simulink model "ISTrain2024"  (R2025a)
settings: Solver=ode4  StartTime=0.0  StopTime=StopTime  FixedStep=StepSize  RelTol=1e-3
undefined symbols (not defined in the file or in its folder): Crr, G, g, LM, LR, m_loco, maxID, maxIQ, maxTorque, mech_eff, Pp, Rr, rw
libraries: slpidlib x3
settings Model: Creator=rafae  LastModifiedBy=mmeni

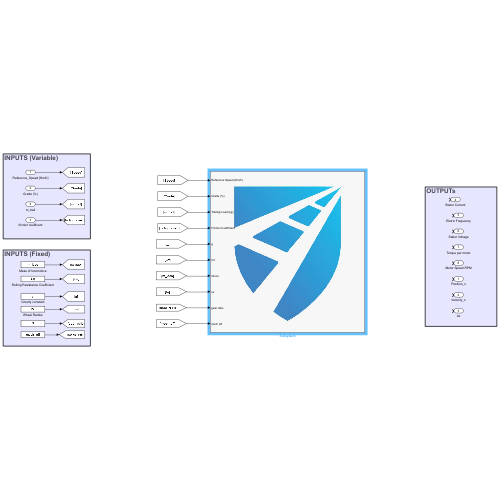
[thumbnail: Simulink's stored preview of the top-level diagram]
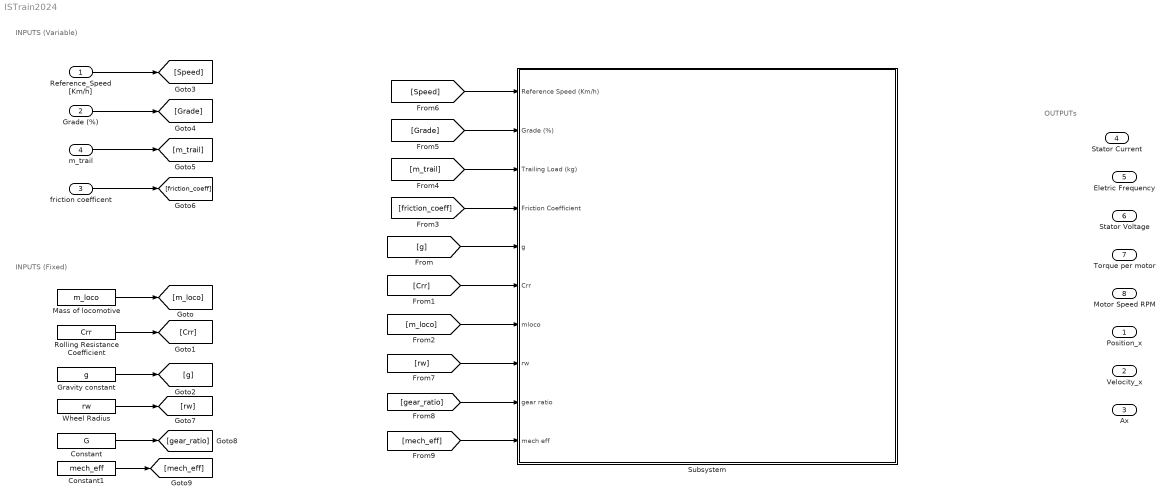
== system ISTrain2024 ==
  note: OUTPUTs
  note: INPUTS (Variable)
  note: INPUTS (Fixed)
  Reference_Speed [Km/h] : Inport
  Grade (%) : Inport  Port=2
  friction coefficent : Inport  Port=3
  m_trail : Inport  Port=4
  Constant : Constant  Value=G
  Constant1 : Constant  Value=mech_eff
  Gravity constant : Constant  Value=g
  Mass of locomotive : Constant  Value=m_loco
  Rolling Resistance Coefficient : Constant  Value=Crr
  Subsystem : Subsystem
      mask Display: image('ist_train_logo.jpg');
  Wheel Radius : Constant  Value=rw
  Position_x : Outport
  Velocity_x : Outport  Port=2
  Ax : Outport  Port=3
  Stator Current : Outport  Port=4
  Eletric Frequency : Outport  Port=5
  Stator Voltage : Outport  Port=6
  Torque per motor : Outport  Port=7
  Motor Speed RPM : Outport  Port=8
  wires:
  Reference_Speed [Km/h]/1 -> [Speed]
  Grade (%)/1 -> [Grade]
  m_trail/1 -> [m_trail]
  friction coefficent/1 -> [friction_coeff]
  Mass of locomotive/1 -> [m_loco]
  Rolling Resistance Coefficient/1 -> [Crr]
  Gravity constant/1 -> [g]
  [g] -> Subsystem/5(g)
  [Crr] -> Subsystem/6(Crr)
  [m_loco] -> Subsystem/7(mloco)
  [friction_coeff] -> Subsystem/4(Friction Coefficient)
  [m_trail] -> Subsystem/3(Trailing Load (kg))
  [Grade] -> Subsystem/2(Grade (%))
  [Speed] -> Subsystem/1(Reference Speed (Km/h))
  Wheel Radius/1 -> [rw]
  [rw] -> Subsystem/8(rw)
  Constant/1 -> [gear_ratio]
  [gear_ratio] -> Subsystem/9(gear ratio)
  Constant1/1 -> [mech_eff]
  [mech_eff] -> Subsystem/10(mech eff)

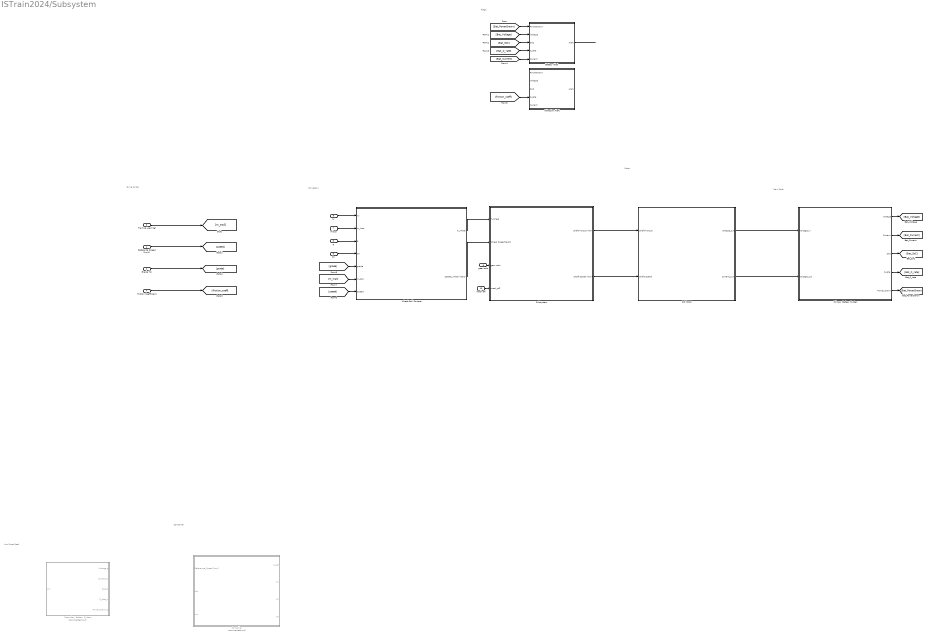
== system ISTrain2024/Subsystem ==
  note: Auxilioar Pack
  note: Drive Cycle
  note: Drivetrain
  note: Motor
  note: Flags
  note: Controller
  note: Main Pack
  Reference Speed (Km/h) : Inport
  Grade (%) : Inport  Port=2
  Trailing Load (kg) : Inport  Port=3
  Friction Coefficient : Inport  Port=4
  g : Inport  Port=5
  Crr : Inport  Port=6
  mloco : Inport  Port=7
  rw : Inport  Port=8
  gear ratio : Inport  Port=9
  mech eff : Inport  Port=10
  Adhesion Alert : Subsystem
      mask Display: image('hazard.jpg');
  Battery Alert : Subsystem
      mask Display: image('hazard.jpg');
  Controller : Subsystem  Commented=on
      mask Display: image('motor controller.jpeg');
  DC Motot : Subsystem
      mask Display: image('motor.jpg');
  Primary Battery Systen : Subsystem
      mask Display: image('battery system.png');
  Secondary Battery System : Subsystem  Commented=on
      mask Display: image('battery system.png');
  Subsystem : Subsystem
      mask Display: image('gear_system.png');
  Wheel-Rail Contact : Subsystem
      mask Display: image('wheel_train.jpg');
  wires:
  Primary Battery Systen/1(Voltage) -> [Bat_Voltage]
  Primary Battery Systen/2(Current) -> [Bat_Current]
  Primary Battery Systen/3(SoC) -> [Bat_SoC]
  Primary Battery Systen/5(Power_drawn) -> [Bat_PowerDrawn]
  Primary Battery Systen/4(C_rate) -> [Bat_C_rate]
  [Bat_Current] -> Battery Alert/5(Current)
  [Bat_C_rate] -> Battery Alert/4(C_rate)
  [Bat_SoC] -> Battery Alert/3(SoC)
  [Bat_Voltage] -> Battery Alert/2(Voltage)
  [Bat_PowerDrawn] -> Battery Alert/1(PowerDrawn)
  Battery Alert/1(Alert) -> ?
  Grade (%)/1 -> [grade]
  Trailing Load (kg)/1 -> [m_trail]
  Friction Coefficient/1 -> [friction_coeff]
  Reference Speed (Km/h)/1 -> [speed]
  g/1 -> Wheel-Rail Contact/3(g)
  Crr/1 -> Wheel-Rail Contact/4(Crr)
  mloco/1 -> Wheel-Rail Contact/2(m_loco)
  [friction_coeff] -> Adhesion Alert/4(C_rate)
  [grade] -> Wheel-Rail Contact/5(grade)
  [m_trail] -> Wheel-Rail Contact/6(m_trail)
  [speed] -> Wheel-Rail Contact/7(Speed)
  rw/1 -> Wheel-Rail Contact/1(rw)
  Wheel-Rail Contact/1(T_wheel) -> Subsystem/1(T_wheel)
  Wheel-Rail Contact/2(Speed_wheel (rad/s)) -> Subsystem/2(Wheel Speed(rad/s))
  gear ratio/1 -> Subsystem/3(gear ratio)
  mech eff/1 -> Subsystem/4(mech_eff)
  Subsystem/1(Shaft Torque (Nm)) -> DC Motot/1(Shaft Torque)
  Subsystem/2(Shaft Speed (rpm)) -> DC Motot/2(Shaft Speed)
  DC Motot/1(Voltage_out) -> Primary Battery Systen/1(Voltage_in)
  DC Motot/2(Current_out) -> Primary Battery Systen/2(Voltage_out)

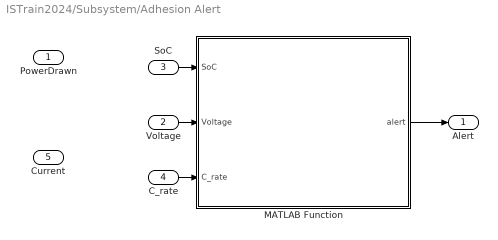
== system ISTrain2024/Subsystem/Adhesion Alert ==
  PowerDrawn : Inport
  Voltage : Inport  Port=2
  SoC : Inport  Port=3
  C_rate : Inport  Port=4
  Current : Inport  Port=5
  MATLAB Function : MATLAB Function  TreatAsAtomicUnit=on
  Alert : Outport
  wires:
  Voltage/1 -> MATLAB Function/2(Voltage)
  SoC/1 -> MATLAB Function/1(SoC)
  MATLAB Function/1(alert) -> Alert/1
  C_rate/1 -> MATLAB Function/3(C_rate)

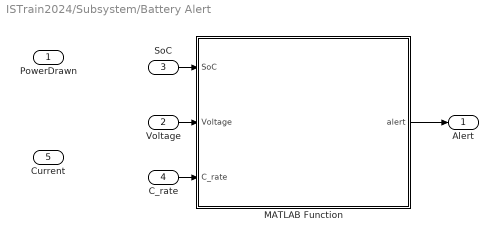
== system ISTrain2024/Subsystem/Battery Alert ==
  PowerDrawn : Inport
  Voltage : Inport  Port=2
  SoC : Inport  Port=3
  C_rate : Inport  Port=4
  Current : Inport  Port=5
  MATLAB Function : MATLAB Function  TreatAsAtomicUnit=on
  Alert : Outport
  wires:
  Voltage/1 -> MATLAB Function/2(Voltage)
  SoC/1 -> MATLAB Function/1(SoC)
  MATLAB Function/1(alert) -> Alert/1
  C_rate/1 -> MATLAB Function/3(C_rate)

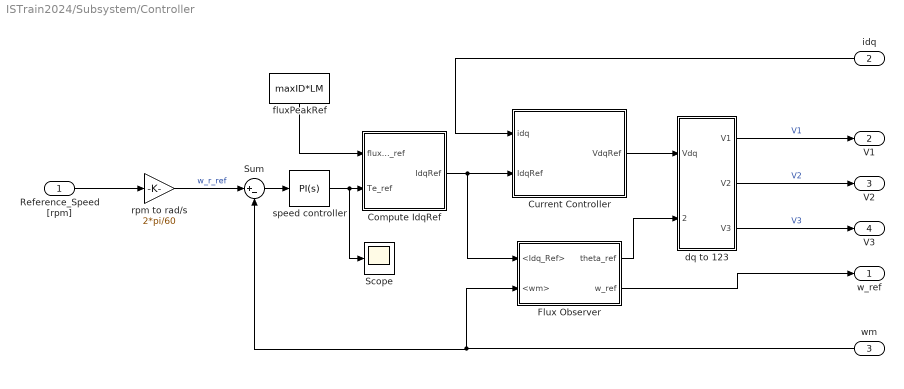
== system ISTrain2024/Subsystem/Controller ==
  Reference_Speed [rpm] : Inport
  idq : Inport  Port=2
  wm : Inport  Port=3
  Compute IdqRef : Subsystem
  Current Controller : Subsystem
  Flux Observer : Subsystem
  Scope : Scope
      settings: ActiveDisplayYMinimum=-8.125  ActiveDisplayYMaximum=73.125
  Sum : Sum  Inputs=|+-
  dq to 123 : Subsystem
  fluxPeakRef : Constant  Value=maxID*LM
  rpm to rad/s : Gain  Gain=2*pi/60
  speed controller : slpidlib/PID Controller  Controller=PI  Form=Parallel  TimeDomain=Continuous-time  UseExternalTs=off  SampleTime=-1  IntegratorMethod=Forward Euler  FilterMethod=Forward Euler  ControllerParametersSource=internal  P=50  I=100  UseKiTs=off  D=0  UseExternalDerivativeSource=off  N=100  UseFilter=on  TunerSelectOption=Transfer Function Based (PID Tuner App)  InitialConditionSource=internal  InitialConditionForIntegrator=0  InitialConditionForFilter=0  DifferentiatorICPrevScaledInput=0  ExternalReset=none  TrackingMode=off  Kt=1  LimitOutput=on  SatLimitsSource=internal  UpperSaturationLimit=maxTorque  LowerSaturationLimit=-maxTorque  LinearizeAsGain=on  AntiWindupMode=back-calculation  Kb=500  LimitIntegrator=off  UpperIntegratorSaturationLimit=inf  LowerIntegratorSaturationLimit=-inf  POutMin=[]  POutMax=[]  IOutMin=[]  IOutMax=[]  DOutMin=[]  DOutMax=[]  NOutMin=[]  NOutMax=[]  SumOutMin=[]  SumOutMax=[]  SaturationOutMin=[]  SaturationOutMax=[]  PParamMin=[]  PParamMax=[]  IParamMin=[]  IParamMax=[]  DParamMin=[]  DParamMax=[]  NParamMin=[]  NParamMax=[]  KbParamMin=[]  KbParamMax=[]  KtParamMin=[]  KtParamMax=[]  KbOutMin=[]  KbOutMax=[]  KtOutMin=[]  KtOutMax=[]  IntegratorOutMin=[]  IntegratorOutMax=[]  FilterOutMin=[]  FilterOutMax=[]  SumI1OutMin=[]  SumI1OutMax=[]  SumI2OutMin=[]  SumI2OutMax=[]  SumI3OutMin=[]  SumI3OutMax=[]  SumI4OutMin=[]  SumI4OutMax=[]  SumDOutMin=[]  SumDOutMax=[]  DifferentiatorOutMin=[]  DifferentiatorOutMax=[]  FilterDiffOutCoefMin=[]  FilterDiffOutCoefMax=[]  ReciprocalOutMin=[]  ReciprocalOutMax=[]  SumDenOutMin=[]  SumDenOutMax=[]  SumNumOutMin=[]  SumNumOutMax=[]  DivideOutMin=[]  DivideOutMax=[]  UdiffTsProdOutMin=[]  UdiffTsProdOutMax=[]  NTsProdOutMin=[]  NTsProdOutMax=[]  UintegralTsProdOutMin=[]  UintegralTsProdOutMax=[]  UngainTsProdOutMin=[]  UngainTsProdOutMax=[]  ClampingZeroOutDataTypeStr=Inherit: Inherit via back propagation  ClampingZeroOutMin=[]  ClampingZeroOutMax=[]  FilterDenConstantOutDataTypeStr=Inherit: Inherit via back propagation  FilterDenConstantOutMin=[]  FilterDenConstantOutMax=[]  PCopyOutDataTypeStr=Inherit: Inherit via back propagation  PCopyOutMin=[]  PCopyOutMax=[]  NCopyOutDataTypeStr=Inherit: Inherit via back propagation  NCopyOutMin=[]  NCopyOutMax=[]  IntegratorContinuousStateAttributes=''  IntegratorStateMustResolveToSignalObject=off  IntegratorRTWStateStorageClass=Auto  FilterContinuousStateAttributes=''  FilterStateMustResolveToSignalObject=off  FilterRTWStateStorageClass=Auto  ParallelPVariant=InternalParameters  IdealPVariant=Disabled  IVariant=InternalParameters  DVariant=Disabled  IntegratorVariant=Continuous  SatVariant=Enabled  AWVariant=BackCalculation  PCopyVariant=Disabled  TRVariant=Disabled  FdbkBlocksVariant=Forward  IdealPFdbkVariant=Disabled  SatFdbkVariant=Disabled  DerivativeFilterVariant=Disabled  NVariant=Disabled  NCopyVariant=Disabled_SignalSpec  FilterICVariant=Disabled  IntegratorICVariant=InternalICs  ExternalResetVariant=Disabled  TRSumVariant=Passthrough  SumFdbkVariant=Disabled  SumVariant=Sum_PI  TsampFilterVariant=InternalTs  TsampNgainVariant=Passthrough  TsampIntegralVariant=Disabled_SignalSpec  ExternalSaturationOutDataTypeStr=Inherit: Same as second input  DerivativeSourceVariant=Disabled  PreIntVariant=InternalPreInt
  w_ref : Outport  VectorParamsAs1DForOutWhenUnconnected=off
  V1 : Outport  Port=2  VectorParamsAs1DForOutWhenUnconnected=off
  V2 : Outport  Port=3  VectorParamsAs1DForOutWhenUnconnected=off
  V3 : Outport  Port=4  VectorParamsAs1DForOutWhenUnconnected=off
  wires:
  Compute IdqRef/1(IdqRef) -> Flux Observer/1(<Idq_Ref>), Current Controller/2(IdqRef)
  Sum/1 -> speed controller/1
  fluxPeakRef/1 -> Compute IdqRef/1(fluxdR_ref)
  dq to 123/3(V3) -> V3/1  "V3"
  wm/1 -> Sum/2, Flux Observer/2(<wm>)
  speed controller/1 -> Scope/1, Compute IdqRef/2(Te_ref)
  idq/1 -> Current Controller/1(idq)
  Reference_Speed [rpm]/1 -> rpm to rad/s/1
  dq to 123/2(V2) -> V2/1  "V2"
  dq to 123/1(V1) -> V1/1  "V1"
  rpm to rad/s/1 -> Sum/1  "w_r_ref"
  Flux Observer/2(w_ref) -> w_ref/1
  Flux Observer/1(theta_ref) -> dq to 123/2(theta_ref)
  Current Controller/1(VdqRef) -> dq to 123/1(Vdq)

== system ISTrain2024/Subsystem/DC Motot ==
  Shaft Torque : Inport
  Shaft Speed : Inport  Port=2
  Voltage_out : Outport
  Current_out : Outport  Port=2

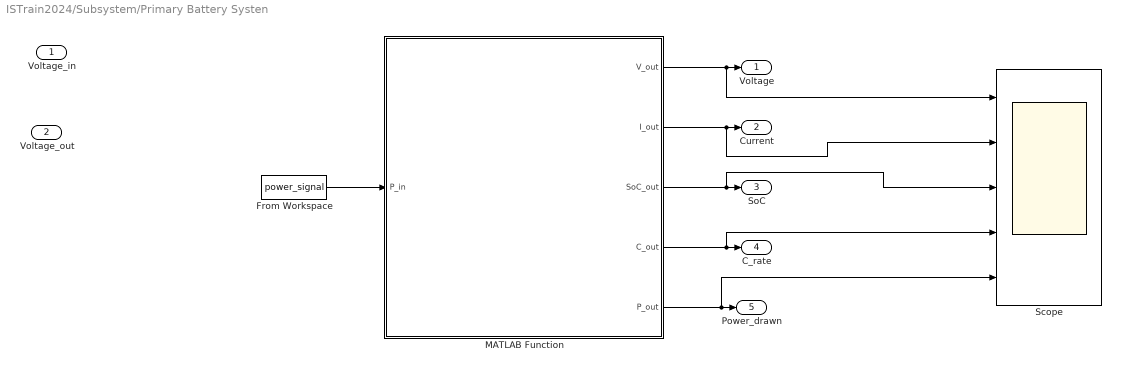
== system ISTrain2024/Subsystem/Primary Battery Systen ==
  Voltage_in : Inport
  Voltage_out : Inport  Port=2
  From Workspace : FromWorkspace  VariableName=power_signal
  MATLAB Function : MATLAB Function  TreatAsAtomicUnit=on
  Scope : Scope  NumInputPorts=5
      settings: ActiveDisplayYMinimum=45.4429  ActiveDisplayYMaximum=52.5661
  Voltage : Outport
  Current : Outport  Port=2
  SoC : Outport  Port=3
  C_rate : Outport  Port=4
  Power_drawn : Outport  Port=5
  wires:
  From Workspace/1 -> MATLAB Function/1(P_in)
  MATLAB Function/1(V_out) -> Scope/1, Voltage/1
  MATLAB Function/2(I_out) -> Scope/2, Current/1
  MATLAB Function/3(SoC_out) -> Scope/3, SoC/1
  MATLAB Function/4(C_out) -> Scope/4, C_rate/1
  MATLAB Function/5(P_out) -> Scope/5, Power_drawn/1

== system ISTrain2024/Subsystem/Secondary Battery System ==
  In1 : Inport
  Voltage_s : Outport
  Current_s : Outport  Port=2
  SoC_s : Outport  Port=3
  C_rate_s : Outport  Port=4
  Power_drawn_s : Outport  Port=5

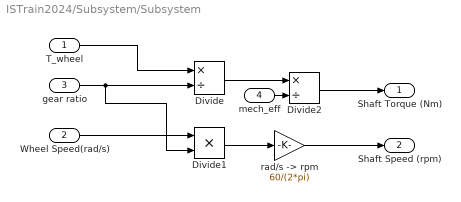
== system ISTrain2024/Subsystem/Subsystem ==
  T_wheel : Inport
  Wheel Speed(rad/s) : Inport  Port=2
  gear ratio : Inport  Port=3
  mech_eff : Inport  Port=4
  Divide : Product  Inputs=*/
  Divide1 : Product  Inputs=**
  Divide2 : Product  Inputs=*/
  "rad/s -> rpm" : Gain  Gain=60/(2*pi)
  Shaft Torque (Nm) : Outport
  Shaft Speed (rpm) : Outport  Port=2
  wires:
  gear ratio/1 -> Divide1/2, Divide/2
  T_wheel/1 -> Divide/1
  Divide/1 -> Divide2/1
  Divide1/1 -> "rad/s -> rpm"/1
  Wheel Speed(rad/s)/1 -> Divide1/1
  "rad/s -> rpm"/1 -> Shaft Speed (rpm)/1
  mech_eff/1 -> Divide2/2
  Divide2/1 -> Shaft Torque (Nm)/1

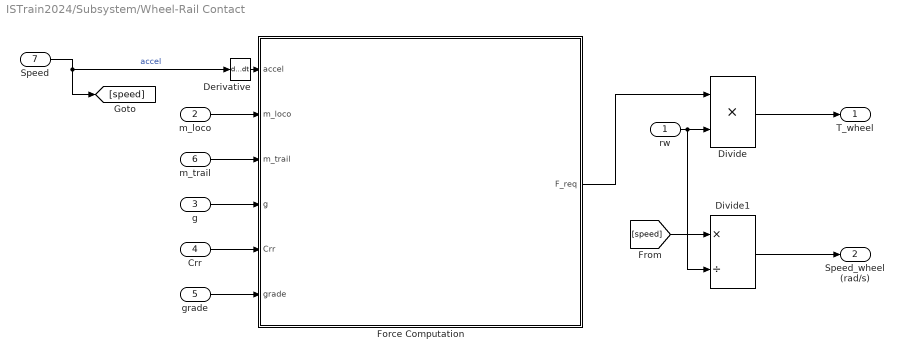
== system ISTrain2024/Subsystem/Wheel-Rail Contact ==
  rw : Inport
  m_loco : Inport  Port=2
  g : Inport  Port=3
  Crr : Inport  Port=4
  grade : Inport  Port=5
  m_trail : Inport  Port=6
  Speed : Inport  Port=7
  Derivative : Derivative
  Divide : Product  Inputs=**
  Divide1 : Product  Inputs=*/
  Force Computation : MATLAB Function  TreatAsAtomicUnit=on
  T_wheel : Outport
  Speed_wheel (rad/s) : Outport  Port=2
  wires:
  g/1 -> Force Computation/4(g)
  m_loco/1 -> Force Computation/2(m_loco)
  Crr/1 -> Force Computation/5(Crr)
  grade/1 -> Force Computation/6(grade)
  m_trail/1 -> Force Computation/3(m_trail)
  Derivative/1 -> Force Computation/1(accel)
  Speed/1 -> Derivative/1, [speed]  "accel"
  rw/1 -> Divide1/2, Divide/2
  Force Computation/1(F_req) -> Divide/1
  Divide/1 -> T_wheel/1
  Divide1/1 -> Speed_wheel (rad/s)/1
  [speed] -> Divide1/1

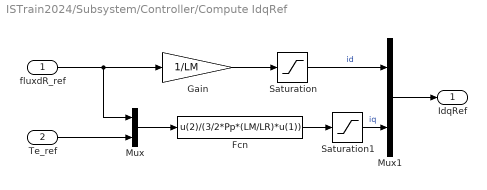
== system ISTrain2024/Subsystem/Controller/Compute IdqRef ==
  fluxdR_ref : Inport
  Te_ref : Inport  Port=2
  Fcn : Fcn  Expr=u(2)/(3/2*Pp*(LM/LR)*u(1))
  Gain : Gain  Gain=1/LM
  Mux : Mux  Inputs=2
  Mux1 : Mux  Inputs=2
  Saturation : Saturate  UpperLimit=maxID  LowerLimit=-maxID
  Saturation1 : Saturate  UpperLimit=maxIQ  LowerLimit=-maxIQ
  IdqRef : Outport  VectorParamsAs1DForOutWhenUnconnected=off
  wires:
  fluxdR_ref/1 -> Mux/1, Gain/1
  Mux/1 -> Fcn/1
  Fcn/1 -> Saturation1/1
  Gain/1 -> Saturation/1
  Mux1/1 -> IdqRef/1
  Te_ref/1 -> Mux/2
  Saturation/1 -> Mux1/1  "id"
  Saturation1/1 -> Mux1/2  "iq"

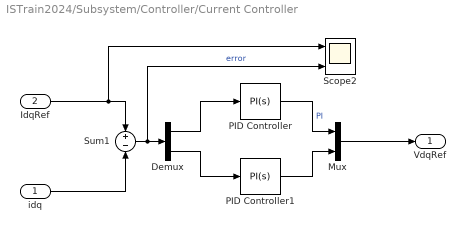
== system ISTrain2024/Subsystem/Controller/Current Controller ==
  idq : Inport
  IdqRef : Inport  Port=2
  Demux : Demux  Outputs=2
  Mux : Mux  Inputs=2
  PID Controller : slpidlib/PID Controller  Controller=PI  Form=Parallel  TimeDomain=Continuous-time  UseExternalTs=off  SampleTime=-1  IntegratorMethod=Forward Euler  FilterMethod=Forward Euler  ControllerParametersSource=internal  P=5  I=100  UseKiTs=off  D=0  UseExternalDerivativeSource=off  N=100  UseFilter=on  TunerSelectOption=Transfer Function Based (PID Tuner App)  InitialConditionSource=internal  InitialConditionForIntegrator=0  InitialConditionForFilter=0  DifferentiatorICPrevScaledInput=0  ExternalReset=none  TrackingMode=off  Kt=1  LimitOutput=on  SatLimitsSource=internal  UpperSaturationLimit=600  LowerSaturationLimit=-600  LinearizeAsGain=on  AntiWindupMode=back-calculation  Kb=1  LimitIntegrator=off  UpperIntegratorSaturationLimit=inf  LowerIntegratorSaturationLimit=-inf  POutMin=[]  POutMax=[]  IOutMin=[]  IOutMax=[]  DOutMin=[]  DOutMax=[]  NOutMin=[]  NOutMax=[]  SumOutMin=[]  SumOutMax=[]  SaturationOutMin=[]  SaturationOutMax=[]  PParamMin=[]  PParamMax=[]  IParamMin=[]  IParamMax=[]  DParamMin=[]  DParamMax=[]  NParamMin=[]  NParamMax=[]  KbParamMin=[]  KbParamMax=[]  KtParamMin=[]  KtParamMax=[]  KbOutMin=[]  KbOutMax=[]  KtOutMin=[]  KtOutMax=[]  IntegratorOutMin=[]  IntegratorOutMax=[]  FilterOutMin=[]  FilterOutMax=[]  SumI1OutMin=[]  SumI1OutMax=[]  SumI2OutMin=[]  SumI2OutMax=[]  SumI3OutMin=[]  SumI3OutMax=[]  SumI4OutMin=[]  SumI4OutMax=[]  SumDOutMin=[]  SumDOutMax=[]  DifferentiatorOutMin=[]  DifferentiatorOutMax=[]  FilterDiffOutCoefMin=[]  FilterDiffOutCoefMax=[]  ReciprocalOutMin=[]  ReciprocalOutMax=[]  SumDenOutMin=[]  SumDenOutMax=[]  SumNumOutMin=[]  SumNumOutMax=[]  DivideOutMin=[]  DivideOutMax=[]  UdiffTsProdOutMin=[]  UdiffTsProdOutMax=[]  NTsProdOutMin=[]  NTsProdOutMax=[]  UintegralTsProdOutMin=[]  UintegralTsProdOutMax=[]  UngainTsProdOutMin=[]  UngainTsProdOutMax=[]  ClampingZeroOutDataTypeStr=Inherit: Inherit via back propagation  ClampingZeroOutMin=[]  ClampingZeroOutMax=[]  FilterDenConstantOutDataTypeStr=Inherit: Inherit via back propagation  FilterDenConstantOutMin=[]  FilterDenConstantOutMax=[]  PCopyOutDataTypeStr=Inherit: Inherit via back propagation  PCopyOutMin=[]  PCopyOutMax=[]  NCopyOutDataTypeStr=Inherit: Inherit via back propagation  NCopyOutMin=[]  NCopyOutMax=[]  IntegratorContinuousStateAttributes=''  IntegratorStateMustResolveToSignalObject=off  IntegratorRTWStateStorageClass=Auto  FilterContinuousStateAttributes=''  FilterStateMustResolveToSignalObject=off  FilterRTWStateStorageClass=Auto  ParallelPVariant=InternalParameters  IdealPVariant=Disabled  IVariant=InternalParameters  DVariant=Disabled  IntegratorVariant=Continuous  SatVariant=Enabled  AWVariant=BackCalculation  PCopyVariant=Disabled  TRVariant=Disabled  FdbkBlocksVariant=Forward  IdealPFdbkVariant=Disabled  SatFdbkVariant=Disabled  DerivativeFilterVariant=Disabled  NVariant=Disabled  NCopyVariant=Disabled_SignalSpec  FilterICVariant=Disabled  IntegratorICVariant=InternalICs  ExternalResetVariant=Disabled  TRSumVariant=Passthrough  SumFdbkVariant=Disabled  SumVariant=Sum_PI  TsampFilterVariant=InternalTs  TsampNgainVariant=Passthrough  TsampIntegralVariant=Disabled_SignalSpec  ExternalSaturationOutDataTypeStr=Inherit: Same as second input  DerivativeSourceVariant=Disabled  PreIntVariant=InternalPreInt
  PID Controller1 : slpidlib/PID Controller  Controller=PI  Form=Parallel  TimeDomain=Continuous-time  UseExternalTs=off  SampleTime=-1  IntegratorMethod=Forward Euler  FilterMethod=Forward Euler  ControllerParametersSource=internal  P=5  I=100  UseKiTs=off  D=0  UseExternalDerivativeSource=off  N=100  UseFilter=on  TunerSelectOption=Transfer Function Based (PID Tuner App)  InitialConditionSource=internal  InitialConditionForIntegrator=0  InitialConditionForFilter=0  DifferentiatorICPrevScaledInput=0  ExternalReset=none  TrackingMode=off  Kt=1  LimitOutput=on  SatLimitsSource=internal  UpperSaturationLimit=600  LowerSaturationLimit=-600  LinearizeAsGain=on  AntiWindupMode=back-calculation  Kb=1  LimitIntegrator=off  UpperIntegratorSaturationLimit=inf  LowerIntegratorSaturationLimit=-inf  POutMin=[]  POutMax=[]  IOutMin=[]  IOutMax=[]  DOutMin=[]  DOutMax=[]  NOutMin=[]  NOutMax=[]  SumOutMin=[]  SumOutMax=[]  SaturationOutMin=[]  SaturationOutMax=[]  PParamMin=[]  PParamMax=[]  IParamMin=[]  IParamMax=[]  DParamMin=[]  DParamMax=[]  NParamMin=[]  NParamMax=[]  KbParamMin=[]  KbParamMax=[]  KtParamMin=[]  KtParamMax=[]  KbOutMin=[]  KbOutMax=[]  KtOutMin=[]  KtOutMax=[]  IntegratorOutMin=[]  IntegratorOutMax=[]  FilterOutMin=[]  FilterOutMax=[]  SumI1OutMin=[]  SumI1OutMax=[]  SumI2OutMin=[]  SumI2OutMax=[]  SumI3OutMin=[]  SumI3OutMax=[]  SumI4OutMin=[]  SumI4OutMax=[]  SumDOutMin=[]  SumDOutMax=[]  DifferentiatorOutMin=[]  DifferentiatorOutMax=[]  FilterDiffOutCoefMin=[]  FilterDiffOutCoefMax=[]  ReciprocalOutMin=[]  ReciprocalOutMax=[]  SumDenOutMin=[]  SumDenOutMax=[]  SumNumOutMin=[]  SumNumOutMax=[]  DivideOutMin=[]  DivideOutMax=[]  UdiffTsProdOutMin=[]  UdiffTsProdOutMax=[]  NTsProdOutMin=[]  NTsProdOutMax=[]  UintegralTsProdOutMin=[]  UintegralTsProdOutMax=[]  UngainTsProdOutMin=[]  UngainTsProdOutMax=[]  ClampingZeroOutDataTypeStr=Inherit: Inherit via back propagation  ClampingZeroOutMin=[]  ClampingZeroOutMax=[]  FilterDenConstantOutDataTypeStr=Inherit: Inherit via back propagation  FilterDenConstantOutMin=[]  FilterDenConstantOutMax=[]  PCopyOutDataTypeStr=Inherit: Inherit via back propagation  PCopyOutMin=[]  PCopyOutMax=[]  NCopyOutDataTypeStr=Inherit: Inherit via back propagation  NCopyOutMin=[]  NCopyOutMax=[]  IntegratorContinuousStateAttributes=''  IntegratorStateMustResolveToSignalObject=off  IntegratorRTWStateStorageClass=Auto  FilterContinuousStateAttributes=''  FilterStateMustResolveToSignalObject=off  FilterRTWStateStorageClass=Auto  ParallelPVariant=InternalParameters  IdealPVariant=Disabled  IVariant=InternalParameters  DVariant=Disabled  IntegratorVariant=Continuous  SatVariant=Enabled  AWVariant=BackCalculation  PCopyVariant=Disabled  TRVariant=Disabled  FdbkBlocksVariant=Forward  IdealPFdbkVariant=Disabled  SatFdbkVariant=Disabled  DerivativeFilterVariant=Disabled  NVariant=Disabled  NCopyVariant=Disabled_SignalSpec  FilterICVariant=Disabled  IntegratorICVariant=InternalICs  ExternalResetVariant=Disabled  TRSumVariant=Passthrough  SumFdbkVariant=Disabled  SumVariant=Sum_PI  TsampFilterVariant=InternalTs  TsampNgainVariant=Passthrough  TsampIntegralVariant=Disabled_SignalSpec  ExternalSaturationOutDataTypeStr=Inherit: Same as second input  DerivativeSourceVariant=Disabled  PreIntVariant=InternalPreInt
  Scope2 : Scope  NumInputPorts=2
      settings: ActiveDisplayYMinimum=-723.5766  ActiveDisplayYMaximum=3684.2345  DataLoggingVariableName=ScopeData3
  Sum1 : Sum  Inputs=+-
  VdqRef : Outport  VectorParamsAs1DForOutWhenUnconnected=off
  wires:
  IdqRef/1 -> Scope2/1, Sum1/1
  idq/1 -> Sum1/2
  PID Controller/1 -> Mux/1  "PI"
  Sum1/1 -> Scope2/2, Demux/1  "error"
  Demux/1 -> PID Controller/1
  Demux/2 -> PID Controller1/1
  PID Controller1/1 -> Mux/2
  Mux/1 -> VdqRef/1

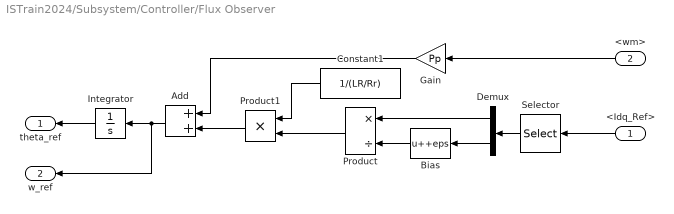
== system ISTrain2024/Subsystem/Controller/Flux Observer ==
  <Idq_Ref> : Inport
  <wm> : Inport  Port=2
  Add : Sum  Inputs=2
  Bias : Bias  Bias=+eps  SaturateOnIntegerOverflow=off
  Constant1 : Constant  Value=1/(LR/Rr)
  Demux : Demux  Outputs=2
  Gain : Gain  Gain=Pp
  Integrator : Integrator
  Product : Product  Inputs=*/
  Product1 : Product
  Selector : Selector  InputPortWidth=2  IndexOptions=Index vector (dialog)  Indices=[2 1]  OutputSizes=1
  theta_ref : Outport  VectorParamsAs1DForOutWhenUnconnected=off
  w_ref : Outport  Port=2  VectorParamsAs1DForOutWhenUnconnected=off
  wires:
  Demux/1 -> Product/1
  <wm>/1 -> Gain/1
  Constant1/1 -> Product1/1
  Selector/1 -> Demux/1
  Product1/1 -> Add/2
  Product/1 -> Product1/2
  <Idq_Ref>/1 -> Selector/1
  Add/1 -> w_ref/1, Integrator/1
  Bias/1 -> Product/2
  Demux/2 -> Bias/1
  Integrator/1 -> theta_ref/1
  Gain/1 -> Add/1

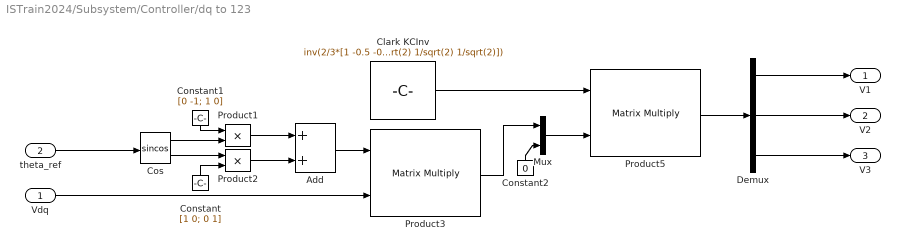
== system ISTrain2024/Subsystem/Controller/dq to 123 ==
  Vdq : Inport
  theta_ref : Inport  Port=2
  Add : Sum
  Clark KCInv : Constant  Value=inv(2/3*[1 -0.5 -0.5; 0 sqrt(3)/2 -sqrt(3)/2; 1/sqrt(2) 1/sqrt(2) 1/sqrt(2)])
  Constant : Constant  Value=[1 0; 0 1]
  Constant1 : Constant  Value=[0 -1; 1 0]
  Constant2 : Constant  Value=0
  Cos : Trigonometry  Operator=sincos
  Demux : Demux  Outputs=3
  Mux : Mux  Inputs=2
  Product1 : Product
  Product2 : Product
  Product3 : Product  Multiplication=Matrix(*)
  Product5 : Product  Multiplication=Matrix(*)
  V1 : Outport  VectorParamsAs1DForOutWhenUnconnected=off
  V2 : Outport  Port=2  VectorParamsAs1DForOutWhenUnconnected=off
  V3 : Outport  Port=3  VectorParamsAs1DForOutWhenUnconnected=off
  wires:
  Cos/1 -> Product1/2
  Constant1/1 -> Product1/1
  Product2/1 -> Add/2
  Cos/2 -> Product2/1
  Product1/1 -> Add/1
  Constant/1 -> Product2/2
  Add/1 -> Product3/1
  Product3/1 -> Mux/1
  Clark KCInv/1 -> Product5/1
  Mux/1 -> Product5/2
  Constant2/1 -> Mux/2
  Vdq/1 -> Product3/2
  Demux/1 -> V1/1
  Demux/2 -> V2/1
  Demux/3 -> V3/1
  Product5/1 -> Demux/1
  theta_ref/1 -> Cos/1

== matlab function ISTrain2024/Subsystem/Battery Alert/MATLAB Function ==
  data: SoC input; alert output; Voltage input; C_rate input
function alert = AlertZone(SoC, Voltage, C_rate)
% Throws an error if any alert condition is violated

% Thresholds
SoC_thresh = 0.10;
V_thresh   = 42;
C_thresh   = 3;

% Check conditions
if SoC < SoC_thresh
    error('ALERT: State of Charge dropped below 10%% (SoC = %.2f)', SoC);
elseif Voltage < V_thresh
    error('ALERT: Voltage dropped below minimum threshold (Voltage = %.2f V)', Voltage);
elseif C_rate > C_thresh
    error('ALERT: C-rate exceeded safe limit (C_rate = %.2f)', C_rate);
end

% No alert
alert = 0;
end

== matlab function ISTrain2024/Subsystem/Primary Battery Systen/MATLAB Function ==
  data: P_in input; V_out output; I_out output; SoC_out output; C_out output; P_out output
function [V_out, I_out, SoC_out, C_out, P_out] = batteryModel(P_in)
% LiFePO4 Battery model (simplified steady-state)
% Assumes constant capacity and internal resistance

% === Parameters ===
persistent SoC_prev V_RC_prev

if isempty(SoC_prev)
    SoC_prev = 1.0;           % initial SoC (100%)
end
if isempty(V_RC_prev)
    V_RC_prev = 0;            % initial RC voltage
end

% Simulation settings
dt = 0.001;                       % 1-second step (adjust to match Simulink sample time)
R0 = 0.02;                    % internal resistance [Ohm]
R1 = 0.005;
C1 = 1000;                    % RC capacitance [F]
voc_min = 42;                 % cut-off voltage [V]

% Battery pack
cell_voltage = 24;            % V
num_series = 2;
num_parallel = 2;
cell_capacity = 100;           % Ah
V_oc_nom = cell_voltage * num_series;
pack_capacity_Ah = cell_capacity * num_parallel;        % 200 Ah
Q_total = pack_capacity_Ah * 3600; % Coulombs

% V_oc vs SoC approximation
SoC_points = linspace(0,1,11);
Voc_points = [24.0 25.2 25.4 25.6 25.7 25.8 25.9 26.0 26.2 26.4 26.8] * num_series;
V_oc = interp1(SoC_points, Voc_points, SoC_prev, 'linear', 'extrap');

% Limit power if voltage or SoC too low
if SoC_prev <= 0.1 || V_oc <= voc_min
    P_in = 0;
end

% Compute current
I = P_in / max(V_oc, 1e-3);

% RC voltage update
dV_RC = (-V_RC_prev + I * R1) / (R1 * C1) * dt;
V_RC_new = V_RC_prev + dV_RC;

% Terminal voltage
V_terminal = V_oc - I * R0 - V_RC_new;
if V_terminal < voc_min
    V_terminal = voc_min;
    I = 0;
    P_in = 0;
end

% Update SoC
dQ = I * dt;
Q_used = (1 - SoC_prev) * Q_total + dQ;
SoC_new = max(0, 1 - Q_used / Q_total);

% Outputs
V_out = V_terminal;
I_out = I;
SoC_out = SoC_new;
C_out = I / pack_capacity_Ah;  % C-rate
P_out = P_in;

% Update persistent vars
SoC_prev = SoC_new;
V_RC_prev = V_RC_new;
end

== matlab function ISTrain2024/Subsystem/Adhesion Alert/MATLAB Function ==
  data: SoC input; alert output; Voltage input; C_rate input
function alert = AlertZone(SoC, Voltage, C_rate)
% Throws an error if any alert condition is violated

% Thresholds
SoC_thresh = 0.10;
V_thresh   = 42;
C_thresh   = 3;

% Check conditions
if SoC < SoC_thresh
    error('ALERT: State of Charge dropped below 10%% (SoC = %.2f)', SoC);
elseif Voltage < V_thresh
    error('ALERT: Voltage dropped below minimum threshold (Voltage = %.2f V)', Voltage);
elseif C_rate > C_thresh
    error('ALERT: C-rate exceeded safe limit (C_rate = %.2f)', C_rate);
end

% No alert
alert = 0;
end

== matlab function ISTrain2024/Subsystem/Wheel-Rail Contact/Force Computation ==
  data: accel input; m_loco input; m_trail input; F_req output; g input; Crr input; grade input
function F_req = Force_Computation(accel, m_loco, m_trail, g, Crr, grade)

a=accel;
m_total=m_trail+m_loco;

F_grade = m_total * g * grade;  % grade
F_rr    = m_total * g * Crr;% rolling
F_a=m_total*a; % Force due to a imposed acceleration
F_req   = F_grade + F_rr+F_a;
end
